simulink model "lab22"  (R2021b)
settings: Solver=VariableStepAuto  StartTime=0.0  StopTime=5  RelTol=1e-3
settings Model: Creator=arek  LastModifiedBy=arek

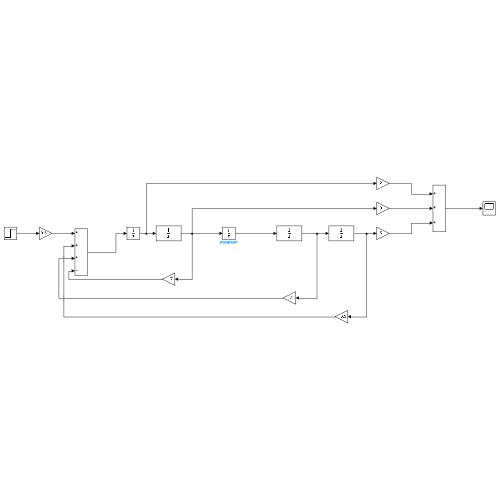
[thumbnail: Simulink's stored preview of the top-level diagram]
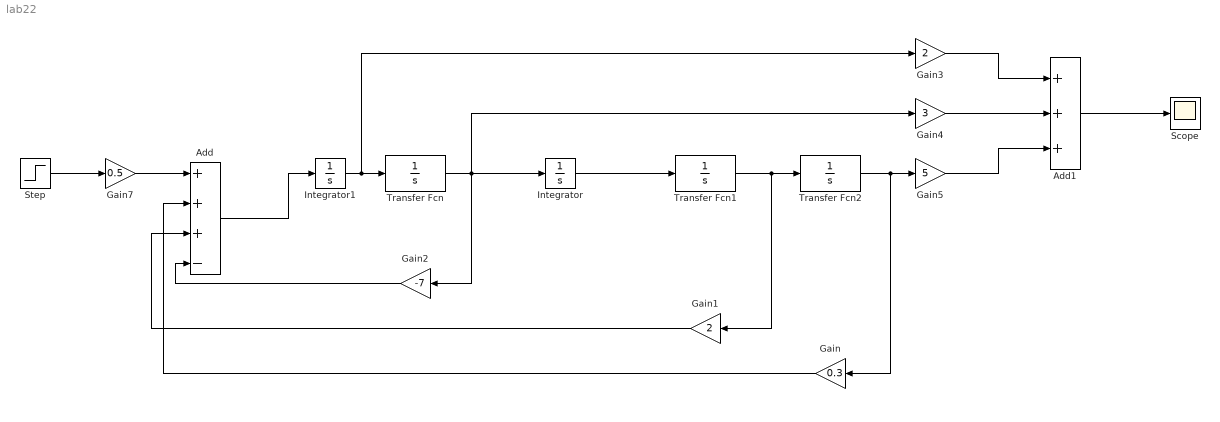
== system lab22 ==
  Add : Sum  Inputs=+++-
  Add1 : Sum  Inputs=+++
  Gain : Gain  Gain=0.3
  Gain1 : Gain  Gain=2
  Gain2 : Gain  Gain=-7
  Gain3 : Gain  Gain=2
  Gain4 : Gain  Gain=3
  Gain5 : Gain  Gain=5
  Gain7 : Gain  Gain=0.5
  Integrator : Integrator
  Integrator1 : Integrator
  Scope : Scope
  Step : Step  SampleTime=0
  Transfer Fcn : TransferFcn  Denominator=[1 0]
  Transfer Fcn1 : TransferFcn  Denominator=[1 0]
  Transfer Fcn2 : TransferFcn  Denominator=[1 0]
  wires:
  Transfer Fcn/1 -> Gain4/1, Gain2/1, Integrator/1
  Transfer Fcn2/1 -> Gain/1, Gain5/1
  Gain3/1 -> Add1/1
  Gain4/1 -> Add1/2
  Gain5/1 -> Add1/3
  Add1/1 -> Scope/1
  Gain/1 -> Add/2
  Gain1/1 -> Add/3
  Gain2/1 -> Add/4
  Transfer Fcn1/1 -> Gain1/1, Transfer Fcn2/1
  Step/1 -> Gain7/1
  Add/1 -> Integrator1/1
  Integrator/1 -> Transfer Fcn1/1
  Integrator1/1 -> Gain3/1, Transfer Fcn/1
  Gain7/1 -> Add/1
